simulink library "THV2THB"  (R2018b)
settings: Solver=ode45  StartTime=0.0  StopTime=10.0  RelTol=1e-3  EnableMultiTasking=on
settings Model: Creator=lena.frank  LastModifiedBy=drhf
settings DataIOCC: LimitDataPoints=on  SaveFormat=Array  SignalLoggingSaveFormat=ModelDataLogs
settings OptimizationCC: ExpressionDepthLimit=2147483647  LifeSpan=inf
settings DebuggingCC: UnderspecifiedInitializationDetection=Classic  MergeDetectMultiDrivingBlocksExec=none  SolverPrmCheckMsg=warning  FcnCallInpInsideContextMsg=warning  StateNameClashWarn=warning  SFUnexpectedBacktrackingDiag=warning  SFNoUnconditionalDefaultTransitionDiag=warning  SFExecutionAtInitializationDiag=none
settings HardwareCC: ProdBitPerPointer=32  ProdBitPerSizeT=32  ProdBitPerPtrDiffT=32  ProdLargestAtomicFloat=None  ProdIntDivRoundTo=Undefined  ProdEndianess=Unspecified  ProdWordSize=32  ProdHWDeviceType=32-bit Generic
settings ModelReferenceCC: PropagateSignalLabelsOutOfModel=off
settings SFSimCC: SimUseLocalCustomCode=off
settings RTWCC: RTWUseLocalCustomCode=off
settings CodeAppCC: StateflowObjectComments=on
settings GRTTargetCC: TargetLangStandard=C89/C90 (ANSI)  GeneratePreprocessorConditionals=Disable all  CombineOutputUpdateFcns=off  GRTInterface=on
settings ConfigComp: CovMetricSettings=dw  CovHtmlReporting=on  CovSaveCumulativeToWorkspaceVar=on  CovSaveSingleToWorkspaceVar=on  CovExternalEMLEnable=off

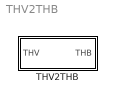
== system THV2THB ==
  THV2THB : Subsystem  InitFcn=load('THB.mat');  mask(THV2THB){}
      mask help: This block converts the old Thermo-Hydraulic-Vector to the Thermo-Hydraulic-Bus.
      mask Help: web(fullfile(path_carnot('help'),'THV2THB.html'),'-helpbrowser')

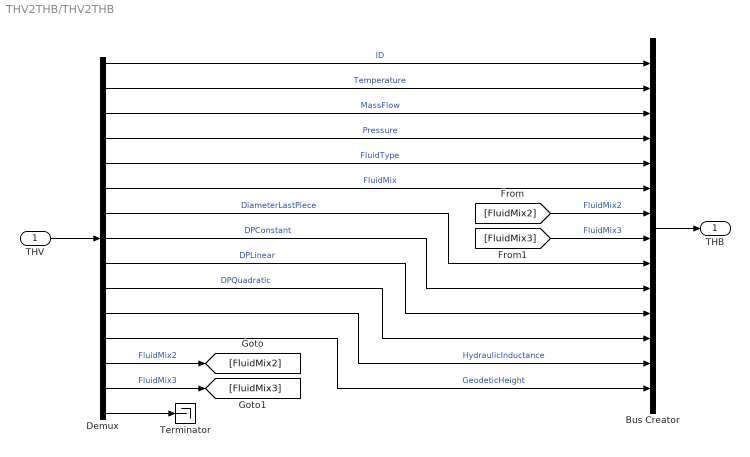
== system THV2THB/THV2THB ==
  THV : Inport
  Bus Creator : BusCreator  Inputs=14  OutDataTypeStr=Bus: THB
  Demux : Demux  Outputs=[1 1 1 1 1 1 1 1 1 1 1 1 1 1 6]
  Terminator : Terminator
  THB : Outport
  wires:
  Demux/11 -> Bus Creator/13  "HydraulicInductance"
  THV/1 -> Demux/1
  Demux/2 -> Bus Creator/2  "Temperature"
  Demux/1 -> Bus Creator/1  "ID"
  Demux/3 -> Bus Creator/3  "MassFlow"
  Demux/4 -> Bus Creator/4  "Pressure"
  Bus Creator/1 -> THB/1
  Demux/5 -> Bus Creator/5  "FluidType"
  Demux/6 -> Bus Creator/6  "FluidMix"
  Demux/7 -> Bus Creator/9  "DiameterLastPiece"
  Demux/8 -> Bus Creator/10  "DPConstant"
  Demux/9 -> Bus Creator/11  "DPLinear"
  Demux/10 -> Bus Creator/12  "DPQuadratic"
  Demux/12 -> Bus Creator/14  "GeodeticHeight"
  Demux/15 -> Terminator/1
  Demux/13 -> [FluidMix2]  "FluidMix2"
  Demux/14 -> [FluidMix3]  "FluidMix3"
  [FluidMix2] -> Bus Creator/7  "FluidMix2"
  [FluidMix3] -> Bus Creator/8  "FluidMix3"
